simulink model "proj1sim"  (R2018b)
settings: Solver=VariableStepAuto  StartTime=0.0  StopTime=.5  RelTol=1e-3
settings Model: Creator=Nick  LastModifiedBy=Nick

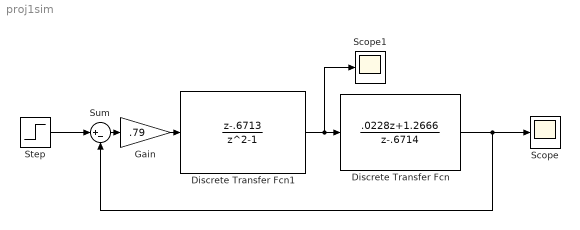
== system proj1sim ==
  Discrete Transfer Fcn : DiscreteTransferFcn  Numerator=[.0228 1.2666]  Denominator=[1 -.6714]  SampleTime=1/50
  Discrete Transfer Fcn1 : DiscreteTransferFcn  Numerator=[1 -.6713]  Denominator="[ 1    0 -1]"
  Gain : Gain  Gain=.79
  Scope : Scope
  Scope1 : Scope
  Step : Step  Time=0  After=2*3.14  SampleTime=0
  Sum : Sum  Inputs=|+-
  wires:
  Step/1 -> Sum/1
  Discrete Transfer Fcn/1 -> Sum/2, Scope/1
  Discrete Transfer Fcn1/1 -> Scope1/1, Discrete Transfer Fcn/1
  Gain/1 -> Discrete Transfer Fcn1/1
  Sum/1 -> Gain/1
